simulink model "AccPed_DoCoordOut"  (R2016b)
settings: configuration reference "CodeGenConfigSet" (kept outside this file)
values from neighbouring files (symbols this model uses):
  AccPed_nMax_C = Calibration.Parameter    [init_AccPed_DoCoordOut.m]    (also in init_AccPed_DoCoordOut_SIL.m = Simulink.Parameter)
  AccPed_nMinBrk_C = Calibration.Parameter    [init_AccPed_DoCoordOut.m]    (also in init_AccPed_DoCoordOut_SIL.m = Simulink.Parameter)
  AccPed_nMinBrkApp_C = Calibration.Parameter    [init_AccPed_DoCoordOut.m]    (also in init_AccPed_DoCoordOut_SIL.m = Simulink.Parameter)
  AccPed_nMinNoBrk_C = Calibration.Parameter    [init_AccPed_DoCoordOut.m]    (also in init_AccPed_DoCoordOut_SIL.m = Simulink.Parameter)
  AccPed_trqLimMax_C = Calibration.Parameter    [init_AccPed_DoCoordOut.m]    (also in init_AccPed_DoCoordOut_SIL.m = Simulink.Parameter)
  COPT_STNSETP_SYSERR_FLT = fi(1,State_uint8)    [init_AccPed_DoCoordOut.m]    (also in init_AccPed_DoCoordOut_SIL.m)
  ENG_N_MAX = fi(6000,EngSpeed_rpm)    [init_AccPed_DoCoordOut.m]    (also in init_AccPed_DoCoordOut_SIL.m)
  ENG_N_MIN = fi(20,EngSpeed_rpm)    [init_AccPed_DoCoordOut.m]    (also in init_AccPed_DoCoordOut_SIL.m)
  TRQPRPHIGH_MAX = fi(3000,Trq_Nm)    [init_AccPed_DoCoordOut.m]    (also in init_AccPed_DoCoordOut_SIL.m)
libraries: CXLib x1
settings Model: Creator=lenovo  LastModifiedBy=bianxuyin
settings ConfigSetRef: SourceLocation=Base Workspace

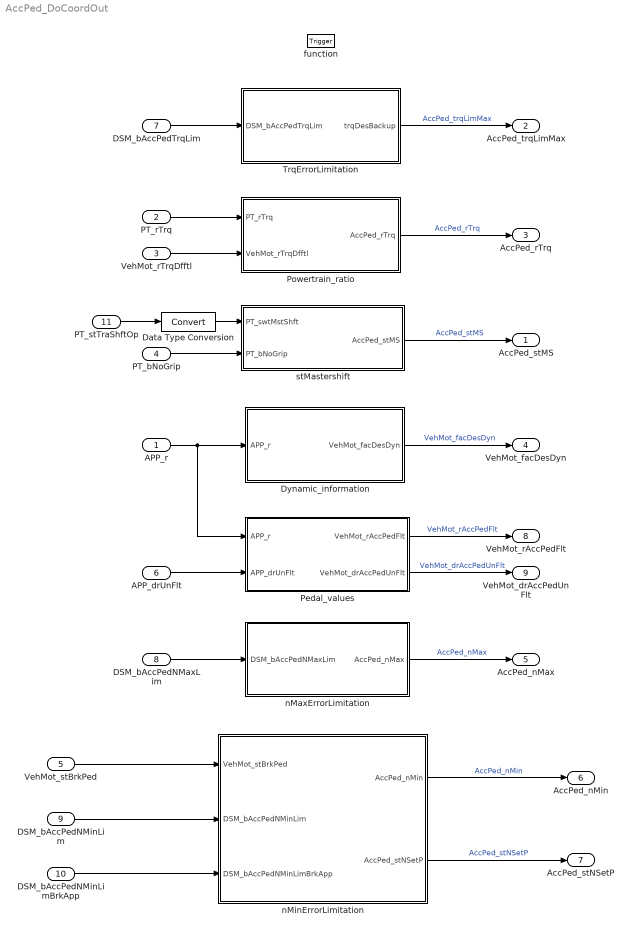
== system AccPed_DoCoordOut ==
  APP_r : Inport  Tag=%  Description=Acceleration pedal sensor 1 value after fault handling  OutMin=0  OutMax=100  OutDataTypeStr=Accpedal_rate
  PT_rTrq : Inport  Description=Powertrain torque ratio  Port=2  OutMin=-100  OutMax=100  OutDataTypeStr=TransRatio
  VehMot_rTrqDfftl : Inport  Description=Torque ratio of differential  Port=3  OutMin=-300  OutMax=300  OutDataTypeStr=TransRatio
  PT_bNoGrip : Inport  Description=Grip reliable exclude  Port=4  OutMin=0  OutMax=1  OutDataTypeStr=boolean
  VehMot_stBrkPed : Inport  Description=Information brake pedal pressed  Port=5  OutMin=0  OutMax=255  OutDataTypeStr=State_uint8
  APP_drUnFlt : Inport  Tag=%/s  Description=Acceleration pedal position gradient of unfilterd value  Port=6  OutMin=-100000  OutMax=100000  OutDataTypeStr=Accpedal_rate_s
  DSM_bAccPedTrqLim : Inport  Description=status of Fid_AccPedTrqLim  Port=7  OutMin=0  OutMax=1  OutDataTypeStr=boolean
  DSM_bAccPedNMaxLim : Inport  Description=status of Fid_AccPedNMaxLim  Port=8  OutMin=0  OutMax=1  OutDataTypeStr=boolean
  DSM_bAccPedNMinLim : Inport  Description=status of Fid_AccPedNMinLim  Port=9  OutMin=0  OutMax=1  OutDataTypeStr=boolean
  DSM_bAccPedNMinLimBrkApp : Inport  Description=status of Fid_AccPedNMinLimBrkApp  Port=10  OutMin=0  OutMax=1  OutDataTypeStr=boolean
  PT_stTraShftOp : Inport  Description=Status if shift operation is active  Port=11  OutMin=0  OutMax=1  OutDataTypeStr=boolean
  function : TriggerPort  TriggerType=function-call  VariantControl=Variant
  Data Type Conversion : DataTypeConversion
  Dynamic_information : Subsystem
  Pedal_values : Subsystem
  Powertrain_ratio : Subsystem
  TrqErrorLimitation : Subsystem
  nMaxErrorLimitation : Subsystem
  nMinErrorLimitation : Subsystem
  "stMastershift " : Subsystem
  AccPed_stMS : Outport  Description=Switch of the mastershift operation  OutMin=0  OutMax=1  OutDataTypeStr=boolean
  AccPed_trqLimMax : Outport  Tag=Nm  Description=Maximum wheel torque in case of accelerator pedal error  Port=2  OutMin=-3000  OutMax=3000  OutDataTypeStr=Trq_Nm
  AccPed_rTrq : Outport  Description=Total drive train ratio of engine - wheel  Port=3  OutMin=-327  OutMax=327  OutDataTypeStr=TransRatio
  VehMot_facDesDyn : Outport  Description=Dynamic factor for driver demand  Port=4  OutMin=-4  OutMax=3.999  OutDataTypeStr=Fact8192
  AccPed_nMax : Outport  Tag=rpm  Description=Maximum engine speed in case of accelerator pedal error  Port=5  OutMin=0  OutMax=6000  OutDataTypeStr=EngSpeed_rpm
  AccPed_nMin : Outport  Tag=rpm  Description=Minimum engine speed in case of accelerator pedal error  Port=6  OutMin=0  OutMax=6000  OutDataTypeStr=EngSpeed_rpm
  AccPed_stNSetP : Outport  Description=Status of engine speed demand of driver demand interpretation  Port=7  OutMin=0  OutMax=255  OutDataTypeStr=State_uint8
  VehMot_rAccPedFlt : Outport  Tag=%  Description=Filtered accelerator pedal value  Port=8  OutMin=0  OutMax=100  OutDataTypeStr=Accpedal_rate
  VehMot_drAccPedUnFlt : Outport  Tag=%/s  Description=accelerator pedal angle slope, unfiltered  Port=9  OutMin=-400  OutMax=399  OutDataTypeStr=Accpedal_rate_s
  wires:
  Dynamic_information/1(VehMot_facDesDyn) -> VehMot_facDesDyn/1  "VehMot_facDesDyn"
  Pedal_values/2(VehMot_drAccPedUnFlt) -> VehMot_drAccPedUnFlt/1  "VehMot_drAccPedUnFlt"
  Pedal_values/1(VehMot_rAccPedFlt) -> VehMot_rAccPedFlt/1  "VehMot_rAccPedFlt"
  APP_drUnFlt/1 -> Pedal_values/2(APP_drUnFlt)
  APP_r/1 -> Pedal_values/1(APP_r), Dynamic_information/1(APP_r)
  nMinErrorLimitation/2(AccPed_stNSetP) -> AccPed_stNSetP/1  "AccPed_stNSetP"
  nMinErrorLimitation/1(AccPed_nMin) -> AccPed_nMin/1  "AccPed_nMin"
  VehMot_stBrkPed/1 -> nMinErrorLimitation/1(VehMot_stBrkPed)
  nMaxErrorLimitation/1(AccPed_nMax) -> AccPed_nMax/1  "AccPed_nMax"
  VehMot_rTrqDfftl/1 -> Powertrain_ratio/2(VehMot_rTrqDfftl)
  PT_rTrq/1 -> Powertrain_ratio/1(PT_rTrq)
  Powertrain_ratio/1(AccPed_rTrq) -> AccPed_rTrq/1  "AccPed_rTrq"
  TrqErrorLimitation/1(trqDesBackup) -> AccPed_trqLimMax/1  "AccPed_trqLimMax"
  DSM_bAccPedTrqLim/1 -> TrqErrorLimitation/1(DSM_bAccPedTrqLim)
  DSM_bAccPedNMaxLim/1 -> nMaxErrorLimitation/1(DSM_bAccPedNMaxLim)
  DSM_bAccPedNMinLim/1 -> nMinErrorLimitation/2(DSM_bAccPedNMinLim)
  DSM_bAccPedNMinLimBrkApp/1 -> nMinErrorLimitation/3(DSM_bAccPedNMinLimBrkApp)
  PT_bNoGrip/1 -> "stMastershift "/2(PT_bNoGrip)
  "stMastershift "/1(AccPed_stMS) -> AccPed_stMS/1  "AccPed_stMS"
  PT_stTraShftOp/1 -> Data Type Conversion/1
  Data Type Conversion/1 -> "stMastershift "/1(PT_swtMstShft)

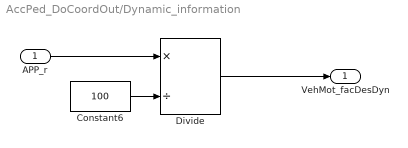
== system AccPed_DoCoordOut/Dynamic_information ==
  APP_r : Inport
  Constant6 : Constant  RequirementInfo={'other' 'APP_requirements.doc' '@Simulink_requirement_item_25' 'true' '手动开关' '' } %GIDa_8c5e3517_ed81_4d84_89e6_6a205131b664  Value=100  OutDataTypeStr=Inherit: Inherit via back propagation
  Divide : Product  Inputs=*/  OutDataTypeStr=Inherit: Inherit via back propagation
  VehMot_facDesDyn : Outport
  wires:
  Divide/1 -> VehMot_facDesDyn/1
  Constant6/1 -> Divide/2
  APP_r/1 -> Divide/1

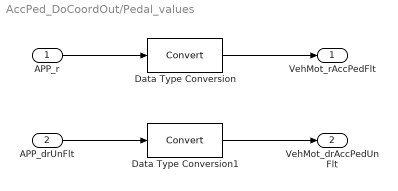
== system AccPed_DoCoordOut/Pedal_values ==
  APP_r : Inport
  APP_drUnFlt : Inport  Port=2
  Data Type Conversion : DataTypeConversion
  Data Type Conversion1 : DataTypeConversion
  VehMot_rAccPedFlt : Outport
  VehMot_drAccPedUnFlt : Outport  Port=2
  wires:
  APP_drUnFlt/1 -> Data Type Conversion1/1
  APP_r/1 -> Data Type Conversion/1
  Data Type Conversion/1 -> VehMot_rAccPedFlt/1
  Data Type Conversion1/1 -> VehMot_drAccPedUnFlt/1

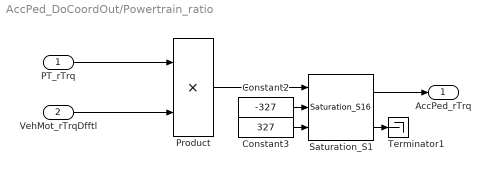
== system AccPed_DoCoordOut/Powertrain_ratio ==
  PT_rTrq : Inport  RequirementInfo={'other' 'APP_requirements.doc' '@Simulink_requirement_item_23' 'true' '振动过滤' '' } %GIDa_6f9ab61e_3782_484b_b3c2_2016ada744a1
  VehMot_rTrqDfftl : Inport  RequirementInfo={'other' 'APP_requirements.doc' '@Simulink_requirement_item_23' 'true' '振动过滤' '' } %GIDa_8ddf94ba_36b5_4edc_8607_0febca9a8724  Port=2
  Constant2 : Constant  Value=-327  OutDataTypeStr=Inherit: Inherit via back propagation
  Constant3 : Constant  Value=327  OutDataTypeStr=Inherit: Inherit via back propagation
  Product : Product  OutDataTypeStr=TransRatio  RndMeth=Round  SaturateOnIntegerOverflow=on
  Saturation_S1 : CXLib/Saturation_S16
  Terminator1 : Terminator
  AccPed_rTrq : Outport
  wires:
  VehMot_rTrqDfftl/1 -> Product/2
  PT_rTrq/1 -> Product/1
  Saturation_S1/2 -> Terminator1/1
  Constant2/1 -> Saturation_S1/2
  Constant3/1 -> Saturation_S1/3
  Product/1 -> Saturation_S1/1
  Saturation_S1/1 -> AccPed_rTrq/1

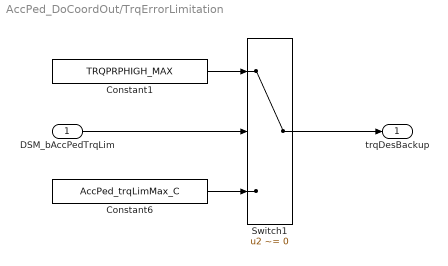
== system AccPed_DoCoordOut/TrqErrorLimitation ==
  DSM_bAccPedTrqLim : Inport  Tag=-  Description=status of Fid_AccPedTrqLim  OutMin=0  OutMax=1  OutDataTypeStr=boolean
  Constant1 : Constant  RequirementInfo={'other' 'APP_requirements.doc' '@Simulink_requirement_item_25' 'true' '手动开关' '' } %GIDa_8f2ea3da_603c_41ca_8fb1_0cbc99bf5789  Value=TRQPRPHIGH_MAX  OutDataTypeStr=Trq_Nm
  Constant6 : Constant  RequirementInfo={'other' 'APP_requirements.doc' '@Simulink_requirement_item_25' 'true' '手动开关' '' } %GIDa_73b9d553_4289_4f10_80ed_fb8748440525  Value=AccPed_trqLimMax_C
  Switch1 : Switch  Criteria=u2 ~= 0  InputSameDT=on
  trqDesBackup : Outport
  wires:
  Constant6/1 -> Switch1/3
  Constant1/1 -> Switch1/1
  Switch1/1 -> trqDesBackup/1
  DSM_bAccPedTrqLim/1 -> Switch1/2

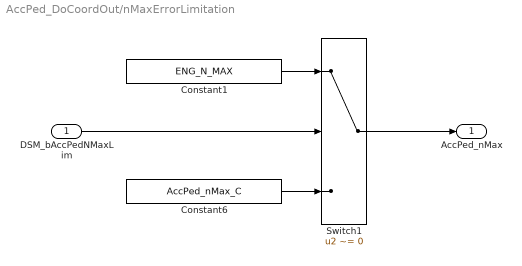
== system AccPed_DoCoordOut/nMaxErrorLimitation ==
  DSM_bAccPedNMaxLim : Inport  Tag=-  Description=status of Fid_AccPedNMaxLim  OutMin=0  OutMax=1  OutDataTypeStr=boolean
  Constant1 : Constant  RequirementInfo={'other' 'APP_requirements.doc' '@Simulink_requirement_item_25' 'true' '手动开关' '' } %GIDa_51055094_ecb6_4dab_8b35_bec466262ea1  Value=ENG_N_MAX  OutDataTypeStr=EngSpeed_rpm
  Constant6 : Constant  RequirementInfo={'other' 'APP_requirements.doc' '@Simulink_requirement_item_25' 'true' '手动开关' '' } %GIDa_73b9d553_4289_4f10_80ed_fb8748440525  Value=AccPed_nMax_C
  Switch1 : Switch  Criteria=u2 ~= 0  InputSameDT=on
  AccPed_nMax : Outport
  wires:
  Constant1/1 -> Switch1/1
  DSM_bAccPedNMaxLim/1 -> Switch1/2
  Switch1/1 -> AccPed_nMax/1
  Constant6/1 -> Switch1/3

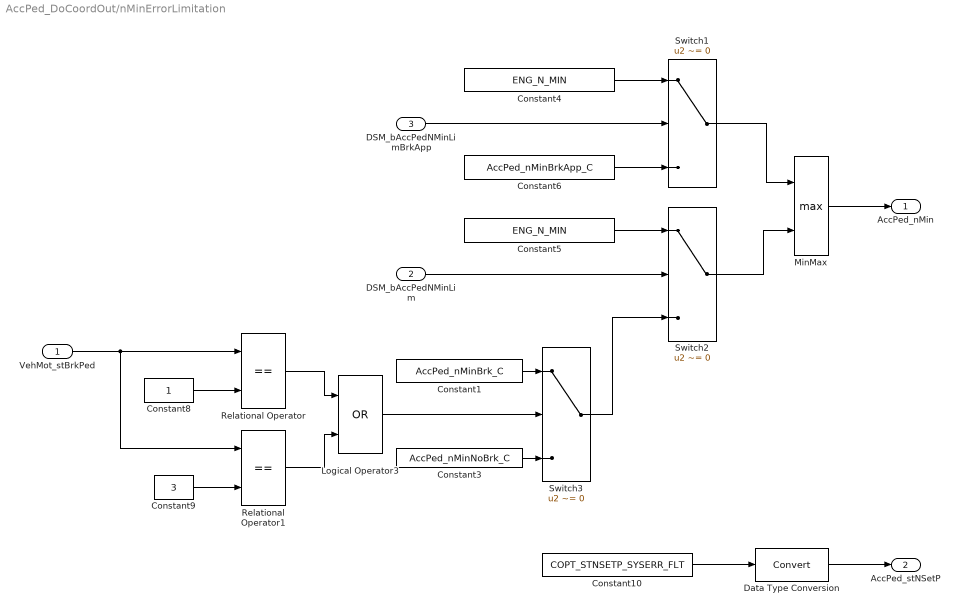
== system AccPed_DoCoordOut/nMinErrorLimitation ==
  VehMot_stBrkPed : Inport
  DSM_bAccPedNMinLim : Inport  Tag=-  Description=status of Fid_AccPedNMinLim  Port=2  OutMin=0  OutMax=1  OutDataTypeStr=boolean
  DSM_bAccPedNMinLimBrkApp : Inport  Tag=-  Description=status of Fid_AccPedNMinLimBrkApp  Port=3  OutMin=0  OutMax=1  OutDataTypeStr=boolean
  Constant1 : Constant  RequirementInfo={'other' 'APP_requirements.doc' '@Simulink_requirement_item_25' 'true' '手动开关' '' } %GIDa_a24f849a_3623_4697_84d1_e2efe02eca1b  Value=AccPed_nMinBrk_C
  Constant10 : Constant  RequirementInfo={'other' 'APP_requirements.doc' '@Simulink_requirement_item_25' 'true' '手动开关' '' } %GIDa_363474ef_ac1a_4efb_b1e8_e5815386ba36  Value=COPT_STNSETP_SYSERR_FLT  OutDataTypeStr=Inherit: Inherit via back propagation
  Constant3 : Constant  RequirementInfo={'other' 'APP_requirements.doc' '@Simulink_requirement_item_25' 'true' '手动开关' '' } %GIDa_fb386ef3_6ef9_4118_925d_70cf957a3a24  Value=AccPed_nMinNoBrk_C
  Constant4 : Constant  RequirementInfo={'other' 'APP_requirements.doc' '@Simulink_requirement_item_25' 'true' '手动开关' '' } %GIDa_61805241_3f6b_4577_aad4_25010caa3789  Value=ENG_N_MIN  OutDataTypeStr=Inherit: Inherit via back propagation
  Constant5 : Constant  RequirementInfo={'other' 'APP_requirements.doc' '@Simulink_requirement_item_25' 'true' '手动开关' '' } %GIDa_a4615913_d4d5_45dc_8b05_77843090dc57  Value=ENG_N_MIN  OutDataTypeStr=Inherit: Inherit via back propagation
  Constant6 : Constant  RequirementInfo={'other' 'APP_requirements.doc' '@Simulink_requirement_item_25' 'true' '手动开关' '' } %GIDa_73b9d553_4289_4f10_80ed_fb8748440525  Value=AccPed_nMinBrkApp_C
  Constant8 : Constant  RequirementInfo={'other' 'APP_requirements.doc' '@Simulink_requirement_item_25' 'true' '手动开关' '' } %GIDa_cb45f827_5d82_4201_b928_bae0d968dab4  OutDataTypeStr=Inherit: Inherit via back propagation
  Constant9 : Constant  RequirementInfo={'other' 'APP_requirements.doc' '@Simulink_requirement_item_25' 'true' '手动开关' '' } %GIDa_cf23e656_9ced_4957_99ef_cbc85a3f777e  Value=3  OutDataTypeStr=Inherit: Inherit via back propagation
  Data Type Conversion : DataTypeConversion
  Logical Operator3 : Logic  Operator=OR  AllPortsSameDT=off  OutDataTypeStr=boolean
  MinMax : MinMax  Function=max  Inputs=2  InputSameDT=on
  Relational Operator : RelationalOperator  Operator===  OutDataTypeStr=boolean  RndMeth=Simplest  InputSameDT=on
  Relational Operator1 : RelationalOperator  Operator===  OutDataTypeStr=boolean  RndMeth=Simplest  InputSameDT=on
  Switch1 : Switch  Criteria=u2 ~= 0  InputSameDT=on
  Switch2 : Switch  Criteria=u2 ~= 0  InputSameDT=on
  Switch3 : Switch  Criteria=u2 ~= 0  InputSameDT=on
  AccPed_nMin : Outport
  AccPed_stNSetP : Outport  Port=2
  wires:
  Constant10/1 -> Data Type Conversion/1
  Constant9/1 -> Relational Operator1/2
  Constant8/1 -> Relational Operator/2
  Constant5/1 -> Switch2/1
  Constant4/1 -> Switch1/1
  MinMax/1 -> AccPed_nMin/1
  Switch2/1 -> MinMax/2
  Switch1/1 -> MinMax/1
  Switch3/1 -> Switch2/3
  Constant3/1 -> Switch3/3
  Constant1/1 -> Switch3/1
  Logical Operator3/1 -> Switch3/2
  Relational Operator1/1 -> Logical Operator3/2
  Relational Operator/1 -> Logical Operator3/1
  VehMot_stBrkPed/1 -> Relational Operator/1, Relational Operator1/1
  DSM_bAccPedNMinLim/1 -> Switch2/2
  DSM_bAccPedNMinLimBrkApp/1 -> Switch1/2
  Constant6/1 -> Switch1/3
  Data Type Conversion/1 -> AccPed_stNSetP/1

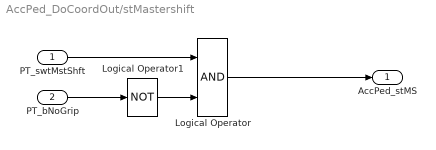
== system AccPed_DoCoordOut/stMastershift  ==
  PT_swtMstShft : Inport  Tag=-  Description=Switch of mastershift state  OutMin=0  OutMax=1  OutDataTypeStr=boolean
  PT_bNoGrip : Inport  Tag=-  Description=Grip reliable exclude  Port=2  OutMin=0  OutMax=1  OutDataTypeStr=boolean
  Logical Operator : Logic  AllPortsSameDT=off  OutDataTypeStr=boolean
  Logical Operator1 : Logic  Operator=NOT  AllPortsSameDT=off  OutDataTypeStr=boolean
  AccPed_stMS : Outport  Tag=-  Description=switch of the mastershift operation  OutMin=0  OutMax=1  OutDataTypeStr=boolean
  wires:
  PT_swtMstShft/1 -> Logical Operator/1
  Logical Operator/1 -> AccPed_stMS/1
  Logical Operator1/1 -> Logical Operator/2
  PT_bNoGrip/1 -> Logical Operator1/1
